simulink model "motorRunner"  (R2017b)
settings: Solver=VariableStepAuto  StartTime=0.0  StopTime=10.0  RelTol=1e-3
libraries: arduinolib x3
settings Model: Creator=Albin  LastModifiedBy=Albin

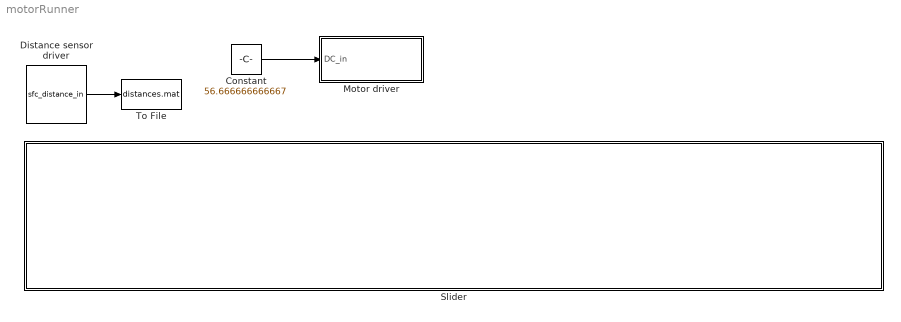
== system motorRunner ==
  Constant : Constant  Value=56.666666666667
  Distance sensor driver : S-Function  InitFcn=try, set_param(gcb,'FunctionName','sfc_distance_in'), end  FunctionName=sfc_distance_in  Parameters=uint8(3),uint8(2)  SFunctionModules=sfc_distance_in_wrapper  SFunctionDeploymentMode=off  EnableBusSupport=off
      mask init:
      | val = [[.9  0.75 0.75 1 1 .9 .9 1]',[1 1 0.75 0.75 .9 .9 1 .9]'];try , sys = get_param(gcb,'SfunBuilderFcnName');if isempty(sys), sys = get_param(gcb,'FunctionName'); end,catch, sys = get_param(gcb,'FunctionName'); end
      settings: CopyFcn=set_param(gcbh,'LinkStatus','none')  PreSaveFcn=try, set_param(gcb,'FunctionName','sfc_distance_in'), end  OpenFcn=sfunctionwizard(gcbh)
      mask Display: plot(val(:,1),val(:,2)),disp(sys), port_label('output',1,'distance')
  Motor driver : Subsystem
  Slider : Subsystem  DialogController=hmiCreateDDGDialog  IsWebBlock=on  mask(MWDashboardBlock){webBlockId=8e1680c4-71f2-4094-8074-d7828c4b90f6, webBlockType=slider, ShowInLibBrowser=on, ShowInitialText=on, HMISrcModelName=untitled}
      mask prompts: webBlockId "WebBlock Id"; webBlockType "WebBlock Type"; HMISrcModelName "Source Model"
      mask help: SimulinkHMI:dialogs:SliderDialogDesc
      mask Help: helpview([docroot '/mapfiles/simulink.map'], 'hmi_slider')
      mask Display:
      | if strcmp(get_param(bdroot(gcb),'BlockDiagramType'), 'library')
      |     image([(matlabroot) '/toolbox/simulink/hmi/icons/Slider.png']);
      | end
  To File : ToFile  Filename=distances.mat  SaveFormat=Timeseries
  wires:
  Distance sensor driver/1 -> To File/1
  Constant/1 -> Motor driver/1(DC_in)

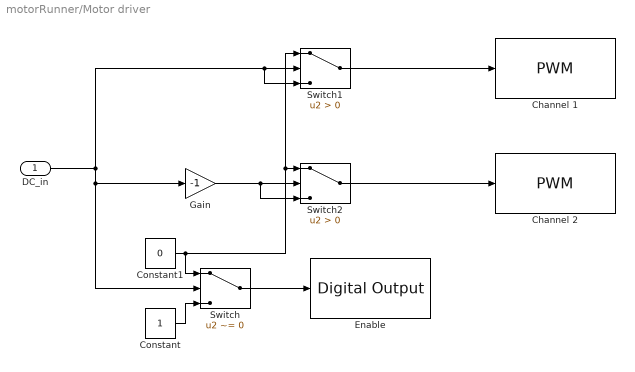
== system motorRunner/Motor driver ==
  DC_in : Inport
  Channel 1 : arduinolib/PWM  pinNumber=10  blockPlatform=arduino
  Channel 2 : arduinolib/PWM  pinNumber=9  blockPlatform=arduino
  Constant : Constant
  Constant1 : Constant  Value=0
  Enable : arduinolib/Digital Output  pinNumber=11  blockPlatform=arduino
  Gain : Gain  Gain=-1
  Switch : Switch  Criteria=u2 ~= 0
  Switch1 : Switch  Criteria=u2 > Threshold
  Switch2 : Switch  Criteria=u2 > Threshold
  wires:
  Constant1/1 -> Switch1/1, Switch2/1, Switch/1
  Constant/1 -> Switch/3
  DC_in/1 -> Switch1/3, Switch1/2, Gain/1, Switch/2
  Switch/1 -> Enable/1
  Switch1/1 -> Channel 1/1
  Switch2/1 -> Channel 2/1
  Gain/1 -> Switch2/3, Switch2/2

== system motorRunner/Slider ==
